simulink model "TP2o"  (R2020a)
settings: Solver=VariableStepAuto  StartTime=0.0  StopTime=10.0  RelTol=1e-3
values from neighbouring files (symbols this model uses):
  K = lqrd(A,B,Q,R)    [TP2.m]
undefined symbols (not defined in the file or in its folder): A, B, C, D, DiscIntNeverNeededParam
settings Model: Creator=João  LastModifiedBy=João

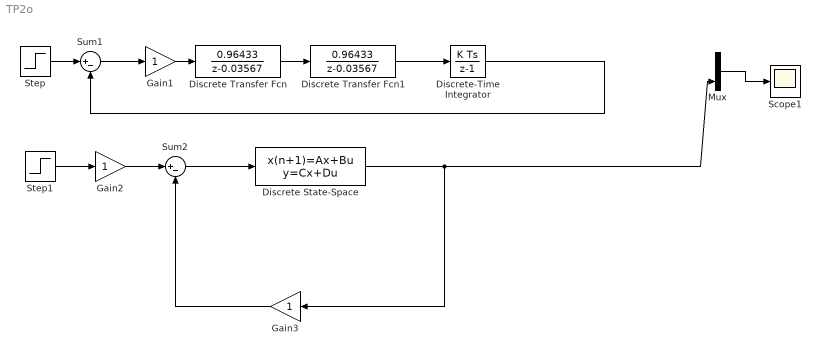
== system TP2o ==
  Discrete Transfer Fcn : DiscreteTransferFcn  Numerator=[0.96433]  Denominator=[1 -0.03567]
  Discrete Transfer Fcn1 : DiscreteTransferFcn  Numerator=[0.96433]  Denominator=[1 -0.03567]
  Discrete State-Space : DiscreteStateSpace  A=(A - B*K)  B=B  C=C  D=D  SampleTime=0.01
  Discrete-Time Integrator : DiscreteIntegrator  SampleTime=-1  ICPrevOutput=DiscIntNeverNeededParam  ICPrevScaledInput=DiscIntNeverNeededParam
  Gain1 : Gain
  Gain2 : Gain
  Gain3 : Gain
  Mux : Mux  Inputs=2
  Scope1 : Scope
  Step : Step  After=10  SampleTime=0
  Step1 : Step  After=10  SampleTime=0
  Sum1 : Sum  Inputs=|+-
  Sum2 : Sum  Inputs=|+-
  wires:
  Step/1 -> Sum1/1
  Mux/1 -> Scope1/1
  Sum1/1 -> Gain1/1
  Gain1/1 -> Discrete Transfer Fcn/1
  Discrete-Time Integrator/1 -> Sum1/2
  Discrete Transfer Fcn/1 -> Discrete Transfer Fcn1/1
  Discrete Transfer Fcn1/1 -> Discrete-Time Integrator/1
  Gain2/1 -> Sum2/1
  Step1/1 -> Gain2/1
  Sum2/1 -> Discrete State-Space/1
  Discrete State-Space/1 -> Gain3/1, Mux/2
  Gain3/1 -> Sum2/2
